simulink model "SWC_FDC_type"  (R2021b)
settings: Solver=FixedStepDiscrete  StartTime=0.0  StopTime=10.0  FixedStep=0.001  RelTol=1e-3
values from neighbouring files (symbols this model uses):
  DID_VCUKey = uint16(0x0202)    [vcu_local_hdr.m]
  DID_XWD = uint16(513)    [vcu_local_hdr.m]
  DIDLen_APSFunConfig = uint16(16)    [vcu_local_hdr.m]
  DIDLen_AutoLock = uint16(1)    [vcu_local_hdr.m]
  DIDLen_DKCKey = uint16(8)    [vcu_local_hdr.m]
  DIDLen_DRLDis = uint16(1)    [vcu_local_hdr.m]
  DIDLen_DynoMode = uint16(1)    [vcu_local_hdr.m]
  DIDLen_FMHTimer = uint16(1)    [vcu_local_hdr.m]
  DIDLen_LFLowPresThre = uint16(1)    [vcu_local_hdr.m]
  DIDLen_LFSensorID = uint16(4)    [vcu_local_hdr.m]
  DIDLen_LRLowPresThre = uint16(1)    [vcu_local_hdr.m]
  DIDLen_LRSensorID = uint16(4)    [vcu_local_hdr.m]
  DIDLen_RFLowPresThre = uint16(1)    [vcu_local_hdr.m]
  DIDLen_RFSensorID = uint16(4)    [vcu_local_hdr.m]
  DIDLen_RRLowPresThre = uint16(1)    [vcu_local_hdr.m]
  DIDLen_RRSensorID = uint16(4)    [vcu_local_hdr.m]
  DIDLen_SensorMode = uint16(1)    [vcu_local_hdr.m]
  DIDLen_TireSize = uint16(16)    [vcu_local_hdr.m]
  DIDLen_TPMSLearnSta = uint16(1)    [vcu_local_hdr.m]
  DIDLen_TurnLampFLThreCurr = uint16(1)    [vcu_local_hdr.m]
  DIDLen_TurnLampFRThreCurr = uint16(1)    [vcu_local_hdr.m]
  DIDLen_TurnLampRLThreCurr = uint16(1)    [vcu_local_hdr.m]
  DIDLen_TurnLampRRThreCurr = uint16(1)    [vcu_local_hdr.m]
  DIDLen_USSConfig = uint16(16)    [vcu_local_hdr.m]
  DIDLen_WhlPres = uint16(4)    [vcu_local_hdr.m]
  DIDLen_WhlSensorBattSta = uint16(1)    [vcu_local_hdr.m]
  DIDLen_WhlTmp = uint16(4)    [vcu_local_hdr.m]
  DIDLen_XWDMode = uint16(1)    [vcu_local_hdr.m]
  DIDNum_APSFunConfig = uint16(0x0903)    [vcu_local_hdr.m]
  DIDNum_AutoLock = uint16(0x0306)    [vcu_local_hdr.m]
  DIDNum_DKCKey = uint16(0x0202)    [vcu_local_hdr.m]
  DIDNum_DRLDis = uint16(0x0307)    [vcu_local_hdr.m]
  DIDNum_DynoMode = uint16(0x0203)    [vcu_local_hdr.m]
  DIDNum_FMHTimer = uint16(0x0305)    [vcu_local_hdr.m]
  DIDNum_LFLowPresThre = uint16(0x0B08)    [vcu_local_hdr.m]
  DIDNum_LFSensorID = uint16(0x0B01)    [vcu_local_hdr.m]
  DIDNum_LRLowPresThre = uint16(0x0B0A)    [vcu_local_hdr.m]
  DIDNum_LRSensorID = uint16(0x0B03)    [vcu_local_hdr.m]
  DIDNum_RFLowPresThre = uint16(0x0B09)    [vcu_local_hdr.m]
  DIDNum_RFSensorID = uint16(0x0B02)    [vcu_local_hdr.m]
  DIDNum_RRLowPresThre = uint16(0x0B0B)    [vcu_local_hdr.m]
  DIDNum_RRSensorID = uint16(0x0B04)    [vcu_local_hdr.m]
  DIDNum_SensorMode = uint16(0x0B0C)    [vcu_local_hdr.m]
  DIDNum_TireSize = uint16(0x0902)    [vcu_local_hdr.m]
  DIDNum_TPMSLearnSta = uint16(0x0B0D)    [vcu_local_hdr.m]
  DIDNum_TurnLampFLThreCurr = uint16(0x0303)    [vcu_local_hdr.m]
  DIDNum_TurnLampFRThreCurr = uint16(0x0301)    [vcu_local_hdr.m]
  DIDNum_TurnLampRLThreCurr = uint16(0x0304)    [vcu_local_hdr.m]
  DIDNum_TurnLampRRThreCurr = uint16(0x0302)    [vcu_local_hdr.m]
  DIDNum_USSConfig = uint16(0x0901)    [vcu_local_hdr.m]
  DIDNum_WhlPres = uint16(0x0B05)    [vcu_local_hdr.m]
  DIDNum_WhlSensorBattSta = uint16(0x0B07)    [vcu_local_hdr.m]
  DIDNum_WhlTmp = uint16(0x0B06)    [vcu_local_hdr.m]
  DIDNum_XWDMode = uint16(0x0201)    [vcu_local_hdr.m]
  DIDVCUKeyLength = uint16(8)    [vcu_local_hdr.m]
  ENUM_DRIVETRAIN_AWD = uint8(  2  )    [vcu_local_hdr.m]
  ENUM_DRIVETRAIN_FWD = uint8(  1  )    [vcu_local_hdr.m]
  ENUM_DRIVETRAIN_RWD = uint8(  0  )    [vcu_local_hdr.m]
  ENUM_TPMSLearnStatus_LEARNED = uint8(  1  )    [vcu_local_hdr.m]
  ENUM_TPMSLearnStatus_LEARNFAIL = uint8(  2  )    [vcu_local_hdr.m]
  ENUM_TPMSLearnStatus_NOTLEARN = uint8(  0  )    [vcu_local_hdr.m]
  ENUM_TPMSSTA_FAT = uint8(  8  )    [vcu_local_hdr.m]
  ENUM_TPMSSTA_LOWBATTERY = uint8(  2  )    [vcu_local_hdr.m]
  FALSE = boolean( 0 )    [vcu_local_hdr.m]
  ONE_INT = uint8(1)    [vcu_local_hdr.m]
  P_boolean = 0.0    [APPTypes.sldd]
  TRUE = boolean( 1 )    [vcu_local_hdr.m]
  ZERO_FLOAT = single(0)    [vcu_local_hdr.m]
  ZERO_INT = uint8(0)    [vcu_local_hdr.m]
undefined symbols (not defined in the file or in its folder): f32_ApsOutVehSpdSig, KHAL_DKCDecryptEnable_flg_ovrdflg, KHAL_DKCDecryptEnable_flg_ovrdval, KHAL_RandomNumberY1_enum, KHAL_RandomNumberY2_enum, KHAL_RandomNumberY_ovrdflg, KHAL_TPMSRESBUTT_flg_ovrdflg, KHAL_TPMSRESBUTT_flg_ovrdval, R_DIDWriteCDD_CSOP_DIDSet_APSFunConfig, R_DIDWriteCDD_CSOP_DIDSet_AutoLock, R_DIDWriteCDD_CSOP_DIDSet_DKCKey, R_DIDWriteCDD_CSOP_DIDSet_DRLDis, R_DIDWriteCDD_CSOP_DIDSet_DynoMode, R_DIDWriteCDD_CSOP_DIDSet_FMHTimer, R_DIDWriteCDD_CSOP_DIDSet_LFLowPresThre, R_DIDWriteCDD_CSOP_DIDSet_LFSensorID, R_DIDWriteCDD_CSOP_DIDSet_LRLowPresThre, R_DIDWriteCDD_CSOP_DIDSet_LRSensorID, R_DIDWriteCDD_CSOP_DIDSet_RFLowPresThre, R_DIDWriteCDD_CSOP_DIDSet_RFSensorID, R_DIDWriteCDD_CSOP_DIDSet_RRLowPresThre, R_DIDWriteCDD_CSOP_DIDSet_RRSensorID, R_DIDWriteCDD_CSOP_DIDSet_SensorMode, R_DIDWriteCDD_CSOP_DIDSet_TireSize, R_DIDWriteCDD_CSOP_DIDSet_TPMSLearnSta, R_DIDWriteCDD_CSOP_DIDSet_TurnLampFLThreCurr, R_DIDWriteCDD_CSOP_DIDSet_TurnLampFRThreCurr, R_DIDWriteCDD_CSOP_DIDSet_TurnLampRLThreCurr, R_DIDWriteCDD_CSOP_DIDSet_TurnLampRRThreCurr, R_DIDWriteCDD_CSOP_DIDSet_USSConfig, R_DIDWriteCDD_CSOP_DIDSet_WhlPres, R_DIDWriteCDD_CSOP_DIDSet_WhlSensorBattSta, R_DIDWriteCDD_CSOP_DIDSet_WhlTmp, R_DIDWriteCDD_CSOP_DIDSet_XWDMode, R_E2E_CAN3_VCU1_CSOP_Write_CAN3_VCU1, R_E2E_CAN3_VCU1_toNIDEC_CSOP_Write_CAN3_VCU1_toNIDEC, R_E2E_CAN4_VCU1_CSOP_Write_CAN4_VCU1, R_FDCCDD_Inner_CSOP_FDC_AppCallSleep, R_HALINCDD_CSOP_PAS_Handler, R_HALINCDD_CSOP_UDS_Main, R_HALOUT_APS_CSOP_ApsOutput, R_HALOUTCDD_CSOP_AppNmStateReq, R_HALOUTCDD_CSOP_SetAcoreRebootCmdACK, R_HALOUTCDD_CSOP_SetSysPwrStat, R_HALOUTCDD_CSOP_SleepRequest, R_IOExpOUT_CDD_CSOP_IOExpSetVal, R_J1939_CAN1_CFGEM1_BAM_CSOP_Write_CAN1_CFGEM1_BAM, R_J1939_CAN1_CFGEM1_DT_CSOP_Write_CAN1_CFGEM1_DT, R_NVMReadCDD_Inner_NVM_ReadOperation, R_NVMWriteCDD_Inner_NVM_WriteOperation, R_UDSCDD_CSOP_DdmRestartOperationCycle, R_WDGCDD_CSOP_Call_Watchdog, R_WDGCDD_CSOP_Call_WDG_AppEnd, R_WDGCDD_CSOP_Call_WDG_AppStart, u16_DIDLen_APSFunConfig, u16_DIDLen_AutoLock, u16_DIDLen_DKCKey, u16_DIDLen_DRLDis, u16_DIDLen_DynoMode, u16_DIDLen_FMHTimer ... (+83)
libraries: simulink x215, FVT_lib x143, hcu_lib x19, hdlsllib x9, app x1, halin x1, halout x1, inp x1, outp x1
(part 2 of 13)

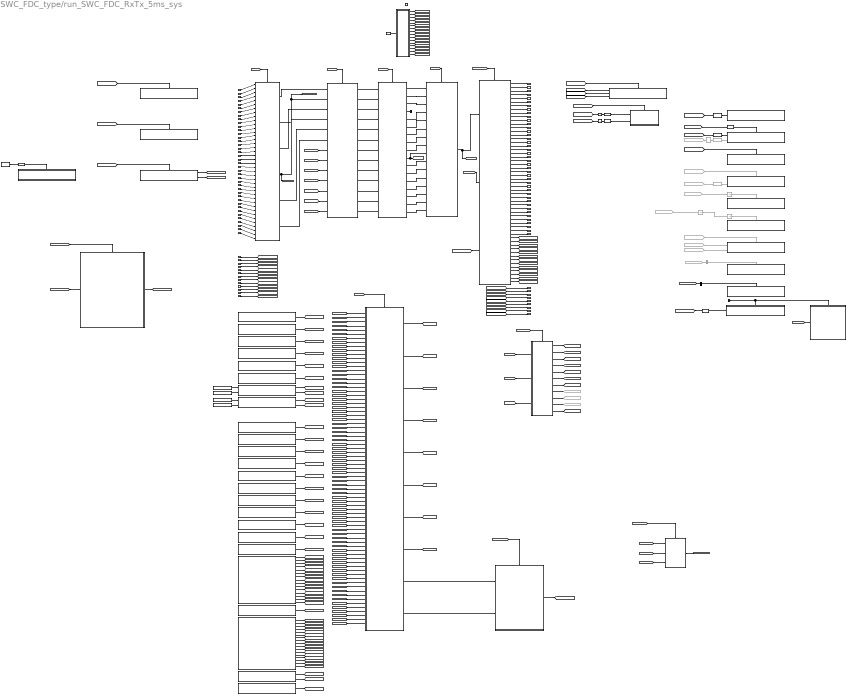
== system SWC_FDC_type/run_SWC_FDC_RxTx_5ms_sys ==
  R_CAN1_DCDC_Status_1_CAN1_SG_DCDC_Status_1_read : Inport
  R_CAN1_DCDC_Status_2_CAN1_SG_DCDC_Status_2_read : Inport  Port=2
  R_CAN1_EAC_Status_1_CAN1_SG_EAC_Status_1_read : Inport  Port=3
  R_CAN1_EBC1_CAN1_SG_EBC1_read : Inport  Port=4
  R_CAN1_EBC2_CAN1_SG_EBC2_read : Inport  Port=5
  R_CAN1_EBC5_CAN1_SG_EBC5_read : Inport  Port=6
  R_CAN1_EHPS_Status_1_CAN1_SG_EHPS_Status_1_read : Inport  Port=7
  R_CAN1_EMC1_EM1_CAN1_SG_EMC1_EM1_read : Inport  Port=8
  R_CAN1_EPB1_CAN1_SG_EPB1_read : Inport  Port=9
  R_CAN1_PDU_Status_1_CAN1_SG_PDU_Status_1_read : Inport  Port=10
  R_CAN2_IVI1_CAN2_SG_IVI1_read : Inport  Port=11
  R_CAN2_IVI2_CAN2_SG_IVI2_read : Inport  Port=12
  R_CAN2_IVI_P20_0_CAN2_SG_IVI_P20_0_read : Inport  Port=13
  R_CAN2_METER1_CAN2_SG_METER1_read : Inport  Port=14
  R_CAN3_BMS1_CAN3_SG_BMS1_read : Inport  Port=15
  R_CAN3_BMS3_CAN3_SG_BMS3_read : Inport  Port=16
  R_CAN3_BMS4_CAN3_SG_BMS4_read : Inport  Port=17
  R_CAN3_BMS5_CAN3_SG_BMS5_read : Inport  Port=18
  R_CAN3_BMS6_CAN3_SG_BMS6_read : Inport  Port=19
  R_CAN3_BMS8_CAN3_SG_BMS8_read : Inport  Port=20
  R_CAN3_CCU1_CAN3_SG_CCU1_read : Inport  Port=21
  R_CAN3_CCU2_CAN3_SG_CCU2_read : Inport  Port=22
  R_CAN3_MCU_B_R1_CAN3_SG_MCU_B_R1_read : Inport  Port=23
  R_CAN3_MCU_B_R2_CAN3_SG_MCU_B_R2_read : Inport  Port=24
  R_CAN3_Shifter1_CAN3_SG_Shifter1_read : Inport  Port=25
  R_CAN4_DKC1_CAN4_SG_DKC1_read : Inport  Port=26
  R_CAN4_DKC2_CAN4_SG_DKC2_read : Inport  Port=27
  R_CAN4_Z24_C1000_0_CAN4_SG_Z24_C1000_0_read : Inport  Port=28
  R_CAN4_Z24_CE100_0_CAN4_SG_Z24_CE100_0_read : Inport  Port=29
  R_CAN4_ZONE_DR1_CAN4_SG_ZONE_DR1_read : Inport  Port=30
  R_CAN4_ZONE_DR_VCU_CAN4_SG_ZONE_DR_VCU_read : Inport  Port=31
  R_CAN4_ZONE_FR1_CAN4_SG_ZONE_FR1_read : Inport  Port=32
  R_CAN4_ZONE_FR_VCU_CAN4_SG_ZONE_FR_VCU_read : Inport  Port=33
  R_CAN4_zGW_APTC1_CAN4_SG_zGW_APTC1_read : Inport  Port=34
  R_CAN4_zGW_CANFr1_CAN4_SG_zGW_CANFr1_read : Inport  Port=35
  R_CAN4_zGW_LINDr1_CAN4_SG_zGW_LINDr1_read : Inport  Port=36
  R_CAN5_TBOX1_CAN5_SG_TBOX1_read : Inport  Port=37
  R_CAN5_TBOX2_CAN5_SG_TBOX2_read : Inport  Port=38
  R_CAN5_TBOX3_CAN5_SG_TBOX3_read : Inport  Port=39
  R_CAN7_Door_Fr1_CAN7_SG_Door_Fr1_read : Inport  Port=40
  IRV_u16Array4_ApsInDist_read : Inport  Port=41
  IRV_u8Array12_ApsInUssSta_read : Inport  Port=42
  IRV_u8Array256_NvmReadArray_read : Inport  Port=43
  IRV_u8Array8_ApsInLevel_read : Inport  Port=44
  IRV_u8Array8_PasInDist_read : Inport  Port=45
  IRV_u8Array9_TPMSData_read : Inport  Port=46
  IRV_u8_ApsInPASChime_read : Inport  Port=47
  IRV_u8_ApsInSensorLayout_read : Inport  Port=48
  IRV_u8_ApsInSysFailSta_read : Inport  Port=49
  IRV_u8_ApsInSysMode_read : Inport  Port=50
  IRV_u8_CTDSW_read : Inport  Port=51
  IRV_u8_TPMSDataInSta_read : Inport  Port=52
  IRV_u8_TrunkHanSW_read : Inport  Port=53
  function : TriggerPort  TriggerType=function-call  VariantControl=(inherit)  SampleTimeType=periodic  SampleTime=-1
  APP : app/APP  SystemSampleTime=-1  VariantActivationTime=update diagram  Latency=0  AutoFrameSizeCalculation=off
  Bus Selector : BusSelector  Commented=on  OutputSignals=VOUTP_EnterNewOperCyc_flg
  Bus Selector1 : BusSelector  OutputSignals=VOUTP_AcoreRebootCmdACK_flg
  Cast To Boolean : DataTypeConversion  OutDataTypeStr=boolean
  Cast To Boolean1 : DataTypeConversion  OutDataTypeStr=boolean
  Constant : Constant  Value=DIDVCUKeyLength
  Constant1 : Constant  Value=DID_VCUKey
  Constant2 : Constant  Value=uint16(ONE_INT)
  Constant3 : Constant  Value=DID_XWD
  Constant4 : Constant  Value=TRUE
  Constant5 : Constant  Value=FALSE
  Constant6 : Constant  Value=ONE_INT
  Data Type Conversion : DataTypeConversion  OutDataTypeStr=uint8
  Data Type Conversion1 : DataTypeConversion  OutDataTypeStr=uint8
  Data Type Conversion2 : DataTypeConversion  Commented=on  OutDataTypeStr=uint8
  Data Type Conversion3 : DataTypeConversion  Commented=on  OutDataTypeStr=uint32
  Data Type Conversion5 : DataTypeConversion  OutDataTypeStr=uint8
  From11 : From  Commented=on  GotoTag=VOUTP_NetworkReq_flg
  From129 : From  Commented=on  GotoTag=BOUTP_outputs
  From14 : From  Commented=on  GotoTag=VOUTP_FdcSlpTime_sec
  From15 : From  Commented=on  GotoTag=VOUTP_FdcSlpReqRisingEdge_flg
  From16 : From  Commented=on  GotoTag=VOUTP_FdcSlpReqRisingEdge_flg
  From17 : From  Commented=on  GotoTag=VOUTP_FdcSlpReqRisingEdge_flg
  From18 : From  Commented=on  GotoTag=Header_Array
  From19 : From  Commented=on  GotoTag=DTC_Array
  From20 : From  Commented=on  GotoTag=DTC_Trigger
  Goto103 : Goto  Commented=on  GotoTag=Header_Array
  Goto108 : Goto  Commented=on  GotoTag=DTC_Array
  Goto116 : Goto  Commented=on  GotoTag=DTC_Trigger
  Ground10 : Ground
  HALOUT_AFTER : Subsystem
  HAL_IN : halin/HAL_IN  SystemSampleTime=-1  VariantActivationTime=update diagram  Latency=0  AutoFrameSizeCalculation=off
  HAL_OUT : halout/HAL_OUT  SystemSampleTime=-1  VariantActivationTime=update diagram  Latency=0  AutoFrameSizeCalculation=off
  Halin_CDD : Subsystem
      settings: RTWSystemCode=Nonreusable function  RTWFcnNameOpts=Use subsystem name  RTWFileNameOpts=Use subsystem name
  INP : inp/INP  SystemSampleTime=-1  VariantActivationTime=update diagram  Latency=0  AutoFrameSizeCalculation=off
  NOT : Logic  Commented=on  Operator=NOT  Inputs=1  AllPortsSameDT=off  OutDataTypeStr=boolean
  OUTP : outp/OUTP  SystemSampleTime=-1  VariantActivationTime=update diagram  Latency=0  AutoFrameSizeCalculation=off
  OUTP_AFTER : Subsystem
      settings: RTWSystemCode=Nonreusable function  RTWFcnNameOpts=Use subsystem name  RTWFileNameOpts=Use subsystem name
  R_FDCCDD_Inner_CSOP_FDC_AppCallSleep : Subsystem
  R_HALINCDD_CSOP_AnyNmID : FunctionCaller  FunctionPrototype=u8_AnyNMID = R_HALINCDD_CSOP_AnyNmID()  OutputArgumentSpecifications=uint8(1)
  R_HALINCDD_CSOP_CAN1BusOff : FunctionCaller  FunctionPrototype=u8_CAN1BusOff = R_HALINCDD_CSOP_CAN1BusOff()  OutputArgumentSpecifications=uint8(1)
  R_HALINCDD_CSOP_CAN2BusOff : FunctionCaller  FunctionPrototype=u8_CAN2BusOff = R_HALINCDD_CSOP_CAN2BusOff()  OutputArgumentSpecifications=uint8(1)
  R_HALINCDD_CSOP_CAN3BusOff : FunctionCaller  FunctionPrototype=u8_CAN3BusOff = R_HALINCDD_CSOP_CAN3BusOff()  OutputArgumentSpecifications=uint8(1)
  R_HALINCDD_CSOP_CAN4BusOff : FunctionCaller  FunctionPrototype=u8_CAN4BusOff = R_HALINCDD_CSOP_CAN4BusOff()  OutputArgumentSpecifications=uint8(1)
  R_HALINCDD_CSOP_CAN5BusOff : FunctionCaller  FunctionPrototype=u8_CAN5BusOff = R_HALINCDD_CSOP_CAN5BusOff()  OutputArgumentSpecifications=uint8(1)
  R_HALINCDD_CSOP_DIDgetDKCdata : FunctionCaller  FunctionPrototype=[u8_DidStaDKC,u8Array8_DidDataDKC] = R_HALINCDD_CSOP_DIDgetDKCdata(u16_lengthDIDDKC,u16_DIDDKC)  InputArgumentSpecifications=uint16(1), uint16(1)  OutputArgumentSpecifications=uint8(1), uint8([1;1;1;1;1;1;1;1])
  R_HALINCDD_CSOP_DIDgetXWDdata : FunctionCaller  FunctionPrototype=[u8_DidStaXWD,u8_DidDataXWD] = R_HALINCDD_CSOP_DIDgetXWDdata(u16_lengthDIDXWD,u16_DIDXWD)  InputArgumentSpecifications=uint16(1), uint16(1)  OutputArgumentSpecifications=uint8(1), uint8(1)
  R_HALINCDD_CSOP_GetAcoreReadyToSleep : FunctionCaller  FunctionPrototype=s8_AcoreReadyToSleep = R_HALINCDD_CSOP_GetAcoreReadyToSleep()  OutputArgumentSpecifications=int8(1)
  R_HALINCDD_CSOP_GetAcoreRebootCmd : FunctionCaller  FunctionPrototype=u8_AcoreRebootCmd = R_HALINCDD_CSOP_GetAcoreRebootCmd()  OutputArgumentSpecifications=uint8(1)
  R_HALINCDD_CSOP_GetAuxBattVoltage : FunctionCaller  FunctionPrototype=u16_AuxBattVol100mV = R_HALINCDD_CSOP_GetAuxBattVoltage()  OutputArgumentSpecifications=uint16(1)
  R_HALINCDD_CSOP_GetBootReason : FunctionCaller  FunctionPrototype=u8_BootReason = R_HALINCDD_CSOP_GetBootReason()  OutputArgumentSpecifications=uint8(1)
  R_HALINCDD_CSOP_GetEvccAplusPwrUpReq : FunctionCaller  FunctionPrototype=u8_EvccAplusPwrUpReq = R_HALINCDD_CSOP_GetEvccAplusPwrUpReq()  OutputArgumentSpecifications=uint8(1)
  R_HALINCDD_CSOP_GetNmState : FunctionCaller  FunctionPrototype=u8_CurrentNMState = R_HALINCDD_CSOP_GetNmState()  OutputArgumentSpecifications=uint8(1)
  R_HALINCDD_CSOP_GetNvmProtectState : FunctionCaller  FunctionPrototype=u8_NvmProtectSta = R_HALINCDD_CSOP_GetNvmProtectState()  OutputArgumentSpecifications=uint8(1)
  R_HALINCDD_CSOP_GetSWID : FunctionCaller  FunctionPrototype=u8Array30_SWID = R_HALINCDD_CSOP_GetSWID()  OutputArgumentSpecifications=uint8([1;1;1;1;1;1;1;1;1;1;1;1;1;1;1;1;1;1;1;1;1;1;1;1;1;1;1;1;1;1])
  R_HALINCDD_CSOP_GetVinpAllowMoveThdOta : FunctionCaller  FunctionPrototype=u8_AllowMovThdOTA = R_HALINCDD_CSOP_GetVinpAllowMoveThdOta()  OutputArgumentSpecifications=uint8(1)
  R_HALINCDD_CSOP_GetVinpPwrReqOta : FunctionCaller  FunctionPrototype=u8_PwrReqOTA = R_HALINCDD_CSOP_GetVinpPwrReqOta()  OutputArgumentSpecifications=uint8(1)
  R_HALINCDD_CSOP_GetWISR : FunctionCaller  FunctionPrototype=u32_WISR = R_HALINCDD_CSOP_GetWISR()  OutputArgumentSpecifications=uint32(1)
  R_HALINCDD_CSOP_HALINCDD_DIRECT : FunctionCaller  FunctionPrototype=[u8_BrakeSW,u8_BrakeLamp,u16_Pedal1Vol,u16_Pedal2Vol,u16_Pedal1Ref5V,u16_Pedal2Ref5V,u8_DrDoorSW,u8_PsDoorSW,u8_RRDoorSW,u8_RLDoorSW,u8_HoodSW,u8_TailgateSW,u8_HazardSW,u8_SeatSW,u8_CrashSignal] = R_HALINCDD_CSOP_HALINCDD_DIRECT()  OutputArgumentSpecifications=uint8(1), uint8(1), uint16(1), uint16(1), uint16(1), uint16(1), uint8(1), uint8(1), uint8(1), uint8(1), uint8(1), uint8(1), uint8(1), uint8(1), uint8(1)
  R_HALINCDD_u8Array4_HWID : FunctionCaller  FunctionPrototype=u8Array4_HWID = R_HALINCDD_u8Array4_HWID()  OutputArgumentSpecifications=uint8([1;1;1;1])
  R_HALIN_APS_CSOP_ApsGetData : FunctionCaller  FunctionPrototype=[u8_GetAPS_Progress_PCT,u8_GetAPS_RQ_Display,u8_GetAPS_SW_Ver,u8_GetAPS_HW_Ver,u8_GetAPS_ExitCondition,f32_GetAPS_Angle_Target,u8_GetAPS_Sta_System,u8_GetAPS_V_Rq_EPAS_Ctrl,u8_GetAPS_Rq_EPAS_Ctrl,u8_GetAPS_Req,f32_GetAPS_DecReq,u8_GetAPS_DecReq_A,f32_GetAPS_SpeedCmd,u8_GetAPS_ShftPosnReq,u8_GetAPS_VMC_Req_A,u8_GetCAAS_Sta,u8_GetCAAS_VMC_Req_A] = R_HALIN_APS_CSOP_ApsGetData()  OutputArgumentSpecifications=uint8(1), uint8(1), uint8(1), uint8(1), uint8(1), single(1), uint8(1), uint8(1), uint8(1), uint8(1), single(1), uint8(1), single(1), uint8(1), uint8(1), uint8(1), uint8(1)
  R_HALIN_IMU_CSOP_IMUGetOffsetVal : Subsystem
  R_HALIN_IMU_CSOP_IMUGetSixAxisVal : FunctionCaller  FunctionPrototype=[s16_IMUSixAxisVal,u8_IMUSixAxisValSta] = R_HALIN_IMU_CSOP_IMUGetSixAxisVal()  OutputArgumentSpecifications=int16([1;1;1;1;1;1]), uint8(1)
  R_HALOUTCDD_CSOP_AppNmStateReq : Subsystem
  R_HALOUTCDD_CSOP_SetAcoreRebootCmdACK : Subsystem
  R_HALOUTCDD_CSOP_SetSysPwrStat : FunctionCaller  FunctionPrototype=R_HALOUTCDD_CSOP_SetSysPwrStat(u8_SysPwrStat)  InputArgumentSpecifications=uint8(1)
  R_HALOUTCDD_CSOP_SleepRequest : Subsystem
  R_NVMReadCDD_Inner_NVM_ReadOperation : Subsystem
  R_NVMWriteCDD_Inner_NVM_WriteOperation : Subsystem
  R_UDSCDD_CSOP_DdmClearDTCNotification : FunctionCaller  FunctionPrototype=u8_ClearDTCcmd = R_UDSCDD_CSOP_DdmClearDTCNotification()  OutputArgumentSpecifications=uint8(1)
  R_UDSCDD_CSOP_DdmRestartOperationCycle : Subsystem
  R_UDSCDD_CSOP_SetDTCStatus : Subsystem
  R_WDGCDD_CSOP_Call_WDG_AppEnd : Subsystem
  R_WDGCDD_CSOP_Call_WDG_AppStart : Subsystem
  R_WDGCDD_CSOP_Call_Watchdog : Subsystem
  Subsystem : Subsystem
  Subsystem1 : Subsystem
  Subsystem2 : Subsystem
  Subsystem3 : Subsystem
  Subsystem4 : Subsystem
  Subsystem5 : Subsystem
  Terminator : Terminator
  Unit Delay : UnitDelay  Commented=on  SampleTime=-1  HasFrameUpgradeWarning=on
  Unit Delay1 : UnitDelay  Commented=on  SampleTime=-1  HasFrameUpgradeWarning=on
  Unit Delay2 : UnitDelay  Commented=on  SampleTime=-1  HasFrameUpgradeWarning=on
  Unit Delay4 : UnitDelay  SampleTime=-1  HasFrameUpgradeWarning=on
  Unit Delay5 : UnitDelay  SampleTime=-1  HasFrameUpgradeWarning=on
  detect_Increase : simulink/Logic and Bit Operations/Detect Increase  vinit=0.0  OutDataTypeStr=boolean
  detect_change : simulink/Logic and Bit Operations/Detect Change  vinit=0  OutDataTypeStr=boolean
  hcu_main_sched : Stateflow chart  TreatAsAtomicUnit=on
  P_CAN1_GW1_C1000_1_CAN1_SG_GW1_C1000_1_write : Outport
  P_CAN2_FD2_CE100_0_CAN2_SG_FD2_CE100_0_write : Outport  Port=2
  P_CAN2_FD2_CE100_1_CAN2_SG_FD2_CE100_1_write : Outport  Port=3
  P_CAN2_FD2_CE200_1_CAN2_SG_FD2_CE200_1_write : Outport  Port=4
  P_CAN3_FD3_BCM1_CAN3_SG_FD3_BCM1_write : Outport  Port=5
  P_CAN3_FD3_THCM2_CAN3_SG_FD3_THCM2_write : Outport  Port=6
  P_CAN3_FD3_V2L1_CAN3_SG_FD3_V2L1_write : Outport  Port=7
  P_CAN3_GW3_CE100_0_CAN3_SG_GW3_CE100_0_write : Outport  Port=8
  P_CAN4_FD4_CE100_1_CAN4_SG_FD4_CE100_1_write : Outport  Port=9
  P_CAN4_FD4_CE100_3_CAN4_SG_FD4_CE100_3_write : Outport  Port=10
  P_CAN4_FD4_CE200_0_CAN4_SG_FD4_CE200_0_write : Outport  Port=11
  P_CAN4_GW4_CE100_0_CAN4_SG_GW4_CE100_0_write : Outport  Port=12
  P_CAN5_FD5_CE100_0_CAN5_SG_FD5_CE100_0_write : Outport  Port=13
  P_CAN5_FD5_Debug1_CAN5_SG_FD5_Debug1_write : Outport  Port=14
  P_CAN5_GW5_CE100_0_CAN5_SG_GW5_CE100_0_write : Outport  Port=15
  P_CAN7_FD7_CE100_0_CAN7_SG_FD7_CE100_0_write : Outport  Port=16
  P_CAN7_FD7_CE100_1_CAN7_SG_FD7_CE100_1_write : Outport  Port=17
  IRV_ms10_CAN1_SG_EMRC1_write : Outport  Port=18  OutDataTypeStr=Bus: DT_CAN1_SG_EMRC1  PortDimensions=1  BusOutputAsStruct=on
  IRV_ms10_CAN1_SG_VCU_PDU_Demand_1_write : Outport  Port=19  OutDataTypeStr=Bus: DT_CAN1_SG_VCU_PDU_Demand_1  PortDimensions=1  BusOutputAsStruct=on
  IRV_ms10_CAN2_SG_GW2_C10_0_write : Outport  Port=20  OutDataTypeStr=Bus: DT_CAN2_SG_GW2_C10_0  PortDimensions=1  BusOutputAsStruct=on
  IRV_ms10_CAN3_SG_FD3_VCU0_write : Outport  Port=21  OutDataTypeStr=Bus: DT_CAN3_SG_FD3_VCU0  PortDimensions=1  BusOutputAsStruct=on
  IRV_ms10_CAN3_SG_FD3_VCU2_write : Outport  Port=22  OutDataTypeStr=Bus: DT_CAN3_SG_FD3_VCU2  PortDimensions=1  BusOutputAsStruct=on
  IRV_ms10_CAN3_SG_FD3_VCU2_toNIDEC_write : Outport  Port=23  OutDataTypeStr=Bus: DT_CAN3_SG_FD3_VCU2_toNIDEC  PortDimensions=1  BusOutputAsStruct=on
  IRV_ms10_CAN3_SG_FD3_VCU5_write : Outport  Port=24  OutDataTypeStr=Bus: DT_CAN3_SG_FD3_VCU5  PortDimensions=1  BusOutputAsStruct=on
  IRV_ms100_CAN1_SG_CCVS_write : Outport  Port=25  OutDataTypeStr=Bus: DT_CAN1_SG_CCVS  PortDimensions=1  BusOutputAsStruct=on
  IRV_ms100_CAN1_SG_FD1_C100_1_write : Outport  Port=26  OutDataTypeStr=Bus: DT_CAN1_SG_FD1_C100_1  PortDimensions=1  BusOutputAsStruct=on
  IRV_ms100_CAN1_SG_FD1_C100_2_write : Outport  Port=27  OutDataTypeStr=Bus: DT_CAN1_SG_FD1_C100_2  PortDimensions=1  BusOutputAsStruct=on
  IRV_ms100_CAN1_SG_FD1_C100_3_write : Outport  Port=28  OutDataTypeStr=Bus: DT_CAN1_SG_FD1_C100_3  PortDimensions=1  BusOutputAsStruct=on
  IRV_ms100_CAN1_SG_FD1_CE100_1_write : Outport  Port=29  OutDataTypeStr=Bus: DT_CAN1_SG_FD1_CE100_1  PortDimensions=1  BusOutputAsStruct=on
  IRV_ms100_CAN1_SG_GW1_C100_4_write : Outport  Port=30  OutDataTypeStr=Bus: DT_CAN1_SG_GW1_C100_4  PortDimensions=1  BusOutputAsStruct=on
  IRV_ms100_CAN2_SG_FD2_C200_1_write : Outport  Port=31  OutDataTypeStr=Bus: DT_CAN2_SG_FD2_C200_1  PortDimensions=1  BusOutputAsStruct=on
  IRV_ms100_CAN3_SG_FD3_THCM1_write : Outport  Port=32  OutDataTypeStr=Bus: DT_CAN3_SG_FD3_THCM1  PortDimensions=1  BusOutputAsStruct=on
  IRV_ms100_CAN4_SG_FD4_C100_0_write : Outport  Port=33  OutDataTypeStr=Bus: DT_CAN4_SG_FD4_C100_0  PortDimensions=1  BusOutputAsStruct=on
  IRV_ms20_CAN2_SG_FD2_C20_0_write : Outport  Port=34  OutDataTypeStr=Bus: DT_CAN2_SG_FD2_C20_0  PortDimensions=1  BusOutputAsStruct=on
  IRV_ms250_CAN1_SG_EEC3_write : Outport  Port=35  OutDataTypeStr=Bus: DT_CAN1_SG_EEC3  PortDimensions=1  BusOutputAsStruct=on
  IRV_ms50_CAN1_SG_EEC2_write : Outport  Port=36  OutDataTypeStr=Bus: DT_CAN1_SG_EEC2  PortDimensions=1  BusOutputAsStruct=on
  IRV_ms50_CAN1_SG_ETC2_write : Outport  Port=37  OutDataTypeStr=Bus: DT_CAN1_SG_ETC2  PortDimensions=1  BusOutputAsStruct=on
  IRV_ms5000_CAN2_SG_FD2_Version_write : Outport  Port=38  OutDataTypeStr=Bus: DT_CAN2_SG_FD2_Version  PortDimensions=1  BusOutputAsStruct=on
  IRV_ms80_CAN1_SG_ETC1_write : Outport  Port=39  OutDataTypeStr=Bus: DT_CAN1_SG_ETC1  PortDimensions=1  BusOutputAsStruct=on
  IRV_E2E_CAN3_SG_FD3_VCU1_write : Outport  Port=40  OutDataTypeStr=Bus: DT_CAN3_SG_FD3_VCU1  PortDimensions=1  BusOutputAsStruct=on
  IRV_E2E_CAN3_SG_FD3_VCU1_toNIDEC_write : Outport  Port=41  OutDataTypeStr=Bus: DT_CAN3_SG_FD3_VCU1_toNIDEC  PortDimensions=1  BusOutputAsStruct=on
  IRV_E2E_CAN4_SG_FD4_CE100_0_write : Outport  Port=42  OutDataTypeStr=Bus: DT_CAN4_SG_FD4_CE100_0  PortDimensions=1  BusOutputAsStruct=on
  IRV_J1939_CAN1_SG_CFGEM1_BAM_write : Outport  Port=43  OutDataTypeStr=Bus: DT_CAN1_SG_CFGEM1_BAM  PortDimensions=1  BusOutputAsStruct=on
  IRV_J1939_CAN1_SG_CFGEM1_DT_write : Outport  Port=44  OutDataTypeStr=Bus: DT_CAN1_SG_CFGEM1_DT  PortDimensions=1  BusOutputAsStruct=on
  IRV_f32_ApsOutVehSpdSig_write : Outport  Port=45  OutDataTypeStr=single  PortDimensions=1
  IRV_u8Array256_NvmWriteArray_write : Outport  Port=46  OutDataTypeStr=uint8  PortDimensions=256
  IRV_u8_ApsOutGearPosnSig_write : Outport  Port=47  OutDataTypeStr=uint8  PortDimensions=1
  IRV_u8_ApsOutSendChrgPlugSta_write : Outport  Port=48  OutDataTypeStr=uint8  PortDimensions=1
  IRV_u8_ApsOutSetFrSensorOnCmd_write : Outport  Port=49  OutDataTypeStr=uint8  PortDimensions=1
  IRV_u8_ApsOutSetFrSensorSwTOCmd_write : Outport  Port=50  OutDataTypeStr=uint8  PortDimensions=1
  IRV_u8_ApsOutSetVehSpdTOCmd_write : Outport  Port=51  OutDataTypeStr=uint8  PortDimensions=1
  wires:
  IRV_u16Array4_ApsInDist_read/1 -> [u16Array4_ApsInDist]
  IRV_u8Array12_ApsInUssSta_read/1 -> [u8Array12_ApsInUssSta]
  IRV_u8Array256_NvmReadArray_read/1 -> [u8Array256_NvmReadArray]
  IRV_u8Array8_ApsInLevel_read/1 -> [u8Array8_ApsInLevel]
  IRV_u8Array8_PasInDist_read/1 -> [u8Array8_PasInDist]
  IRV_u8Array9_TPMSData_read/1 -> [u8Array9_TPMSData]
  IRV_u8_ApsInPASChime_read/1 -> [u8_ApsInPASChime]
  IRV_u8_ApsInSensorLayout_read/1 -> [u8_ApsInSensorLayout]
  IRV_u8_ApsInSysFailSta_read/1 -> [u8_ApsInSysFailSta]
  IRV_u8_ApsInSysMode_read/1 -> [u8_ApsInSysMode]
  IRV_u8_CTDSW_read/1 -> [u8_CTDSW]
  IRV_u8_TPMSDataInSta_read/1 -> [u8_TPMSDataInSta]
  IRV_u8_TrunkHanSW_read/1 -> [u8_TrunkHanSW]
  [J1939_CAN1_SG_CFGEM1_BAM] -> IRV_J1939_CAN1_SG_CFGEM1_BAM_write/1
  [J1939_CAN1_SG_CFGEM1_DT] -> IRV_J1939_CAN1_SG_CFGEM1_DT_write/1
  [f32_ApsOutVehSpdSig] -> IRV_f32_ApsOutVehSpdSig_write/1
  [u8Array256_NvmWriteArray] -> IRV_u8Array256_NvmWriteArray_write/1
  [u8_ApsOutGearPosnSig] -> IRV_u8_ApsOutGearPosnSig_write/1
  [u8_ApsOutSendChrgPlugSta] -> IRV_u8_ApsOutSendChrgPlugSta_write/1
  [u8_ApsOutSetFrSensorOnCmd] -> IRV_u8_ApsOutSetFrSensorOnCmd_write/1
  [u8_ApsOutSetFrSensorSwTOCmd] -> IRV_u8_ApsOutSetFrSensorSwTOCmd_write/1
  [u8_ApsOutSetVehSpdTOCmd] -> IRV_u8_ApsOutSetVehSpdTOCmd_write/1
  R_HALINCDD_CSOP_AnyNmID/1 -> [u8_AnyNMID]
  R_HALINCDD_CSOP_CAN1BusOff/1 -> [u8_CAN1BusOff]
  R_HALINCDD_CSOP_CAN2BusOff/1 -> [u8_CAN2BusOff]
  R_HALINCDD_CSOP_CAN3BusOff/1 -> [u8_CAN3BusOff]
  R_HALINCDD_CSOP_CAN4BusOff/1 -> [u8_CAN4BusOff]
  R_HALINCDD_CSOP_CAN5BusOff/1 -> [u8_CAN5BusOff]
  Constant/1 -> R_HALINCDD_CSOP_DIDgetDKCdata/1
  Constant1/1 -> R_HALINCDD_CSOP_DIDgetDKCdata/2
  R_HALINCDD_CSOP_DIDgetDKCdata/1 -> [u8_DidStaDKC]
  R_HALINCDD_CSOP_DIDgetDKCdata/2 -> [u8Array8_DidDataDKC]
  Constant2/1 -> R_HALINCDD_CSOP_DIDgetXWDdata/1
  Constant3/1 -> R_HALINCDD_CSOP_DIDgetXWDdata/2
  R_HALINCDD_CSOP_DIDgetXWDdata/1 -> [u8_DidStaXWD]
  R_HALINCDD_CSOP_DIDgetXWDdata/2 -> [u8_DidDataXWD]
  R_HALINCDD_CSOP_GetAcoreReadyToSleep/1 -> [s8_AcoreReadyToSleep]
  R_HALINCDD_CSOP_GetAcoreRebootCmd/1 -> [u8_AcoreRebootCmd]
  R_HALINCDD_CSOP_GetAuxBattVoltage/1 -> [u16_AuxBattVol100mV]
  R_HALINCDD_CSOP_GetBootReason/1 -> [u8_BootReason]
  R_HALINCDD_CSOP_GetEvccAplusPwrUpReq/1 -> [u8_EvccAplusPwrUpReq]
  R_HALINCDD_CSOP_GetNmState/1 -> [u8_CurrentNMState]
  R_HALINCDD_CSOP_GetNvmProtectState/1 -> [u8_NvmProtectSta]
  R_HALINCDD_CSOP_GetSWID/1 -> [u8Array30_SWID]
  R_HALINCDD_CSOP_GetVinpAllowMoveThdOta/1 -> [u8_AllowMovThdOTA]
  R_HALINCDD_CSOP_GetVinpPwrReqOta/1 -> [u8_PwrReqOTA]
  R_HALINCDD_CSOP_GetWISR/1 -> [u32_WISR]
  R_HALINCDD_CSOP_HALINCDD_DIRECT/1 -> [u8_BrakeSW]
  R_HALINCDD_CSOP_HALINCDD_DIRECT/2 -> [u8_BrakeLamp]
  R_HALINCDD_CSOP_HALINCDD_DIRECT/3 -> [u16_Pedal1Vol]
  R_HALINCDD_CSOP_HALINCDD_DIRECT/4 -> [u16_Pedal2Vol]
  R_HALINCDD_CSOP_HALINCDD_DIRECT/5 -> [u16_Pedal1Ref5V]
  R_HALINCDD_CSOP_HALINCDD_DIRECT/6 -> [u16_Pedal2Ref5V]
  R_HALINCDD_CSOP_HALINCDD_DIRECT/7 -> [u8_DrDoorSW]
  R_HALINCDD_CSOP_HALINCDD_DIRECT/8 -> [u8_PsDoorSW]
  R_HALINCDD_CSOP_HALINCDD_DIRECT/9 -> [u8_RRDoorSW]
  R_HALINCDD_CSOP_HALINCDD_DIRECT/10 -> [u8_RLDoorSW]
  R_HALINCDD_CSOP_HALINCDD_DIRECT/11 -> [u8_HoodSW]
  R_HALINCDD_CSOP_HALINCDD_DIRECT/12 -> [u8_TailgateSW]
  R_HALINCDD_CSOP_HALINCDD_DIRECT/13 -> [u8_HazardSW]
  R_HALINCDD_CSOP_HALINCDD_DIRECT/14 -> [u8_SeatSW]
  R_HALINCDD_CSOP_HALINCDD_DIRECT/15 -> [u8_CrashSignal]
  R_HALINCDD_u8Array4_HWID/1 -> [u8Array4_HWID]
  R_HALIN_APS_CSOP_ApsGetData/1 -> [u8_GetAPS_Progress_PCT]
  R_HALIN_APS_CSOP_ApsGetData/2 -> [u8_GetAPS_RQ_Display]
  R_HALIN_APS_CSOP_ApsGetData/3 -> [u8_GetAPS_SW_Ver]
  R_HALIN_APS_CSOP_ApsGetData/4 -> [u8_GetAPS_HW_Ver]
  R_HALIN_APS_CSOP_ApsGetData/5 -> [u8_GetAPS_ExitCondition]
  R_HALIN_APS_CSOP_ApsGetData/6 -> [f32_GetAPS_Angle_Target]
  R_HALIN_APS_CSOP_ApsGetData/7 -> [u8_GetAPS_Sta_System]
  R_HALIN_APS_CSOP_ApsGetData/8 -> [u8_GetAPS_V_Rq_EPAS_Ctrl]
  R_HALIN_APS_CSOP_ApsGetData/9 -> [u8_GetAPS_Rq_EPAS_Ctrl]
  R_HALIN_APS_CSOP_ApsGetData/10 -> [u8_GetAPS_Req]
  R_HALIN_APS_CSOP_ApsGetData/11 -> [f32_GetAPS_DecReq]
  R_HALIN_APS_CSOP_ApsGetData/12 -> [u8_GetAPS_DecReq_A]
  R_HALIN_APS_CSOP_ApsGetData/13 -> [f32_GetAPS_SpeedCmd]
  R_HALIN_APS_CSOP_ApsGetData/14 -> [u8_GetAPS_ShftPosnReq]
  R_HALIN_APS_CSOP_ApsGetData/15 -> [u8_GetAPS_VMC_Req_A]
  R_HALIN_APS_CSOP_ApsGetData/16 -> [u8_GetCAAS_Sta]
  R_HALIN_APS_CSOP_ApsGetData/17 -> [u8_GetCAAS_VMC_Req_A]
  R_HALIN_IMU_CSOP_IMUGetSixAxisVal/1 -> [s16_IMUSixAxisVal]
  R_HALIN_IMU_CSOP_IMUGetSixAxisVal/2 -> [u8_IMUSixAxisValSta]
  R_UDSCDD_CSOP_DdmClearDTCNotification/1 -> [u8_ClearDTCcmd]
  Data Type Conversion/1 -> R_HALOUTCDD_CSOP_SetSysPwrStat/1
  [VOUTP_SysPowerMode_enum] -> Data Type Conversion/1
  Data Type Conversion1/1 -> R_HALOUTCDD_CSOP_AppNmStateReq/1(WakeReq)
  [VOUTP_NetworkReq_flg] -> Data Type Conversion1/1
  Data Type Conversion2/1 -> R_HALOUTCDD_CSOP_AppNmStateReq/2(SleepReq)
  NOT/1 -> Data Type Conversion2/1
  From11/1 -> NOT/1
  detect_change/1 -> R_HALOUTCDD_CSOP_AppNmStateReq/Enable
  [VOUTP_NetworkReq_flg] -> detect_change/1
  [VOUTP_NvWriteReqRisingEdge_flg] -> R_NVMWriteCDD_Inner_NVM_WriteOperation/Enable
  Data Type Conversion3/1 -> R_HALOUTCDD_CSOP_SleepRequest/2(WakeUpTime)
  From14/1 -> Data Type Conversion3/1
  From15/1 -> R_HALOUTCDD_CSOP_SleepRequest/Enable
  Unit Delay/1 -> R_WDGCDD_CSOP_Call_WDG_AppEnd/Enable
  From16/1 -> Unit Delay/1
  Unit Delay1/1 -> R_FDCCDD_Inner_CSOP_FDC_AppCallSleep/Enable
  Unit Delay2/1 -> Unit Delay1/1
  From17/1 -> Unit Delay2/1
  From18/1 -> R_UDSCDD_CSOP_SetDTCStatus/1(Header_Array)
  From19/1 -> R_UDSCDD_CSOP_SetDTCStatus/2(DTC_Array)
  From20/1 -> R_UDSCDD_CSOP_SetDTCStatus/Enable
  [trig_Read_NVM_00] -> R_NVMReadCDD_Inner_NVM_ReadOperation/Trigger
  [trig_WDG] -> R_WDGCDD_CSOP_Call_Watchdog/Trigger
  detect_Increase/1 -> R_WDGCDD_CSOP_Call_WDG_AppStart/Enable
  Constant4/1 -> detect_Increase/1
  [trig_ReadIMUOffset_00] -> R_HALIN_IMU_CSOP_IMUGetOffsetVal/Trigger
  R_HALIN_IMU_CSOP_IMUGetOffsetVal/1(Out1) -> [s16_IMUOffsetVal]
  R_HALIN_IMU_CSOP_IMUGetOffsetVal/2(Out2) -> [u8_IMUOffsetValSta]
  [E2E_CAN3_VCU1_Trigger] -> HALOUT_AFTER/1(E2E_CAN3_VCU1_Trigger)
  [E2E_CAN3_VCU1_toNIDEC_Trigger] -> HALOUT_AFTER/2(E2E_CAN3_VCU1_Trigger_toNIDEC)
  [E2E_CAN4_VCU1_Trigger] -> HALOUT_AFTER/3(E2E_CAN4_VCU1_Trigger)
  [trig_HAL_OUTAFTER_50_1] -> HALOUT_AFTER/Trigger
  INP/5 -> APP/5
  INP/1 -> APP/1
  hcu_main_sched/12(trig_OUTP_40()) -> [trig_OUTP_40]
  hcu_main_sched/5(trig_GetDID()) -> [trig_GetDID]
  hcu_main_sched/10(trig_INP_20()) -> [trig_INP_20]
  APP/10 -> OUTP/9, [BSCP_outputs]
  INP/11 -> APP/11
  hcu_main_sched/6(trig_HAL_IN_10()) -> [trig_HAL_IN_10]
  Constant5/1 -> hcu_main_sched/1(VHAL_FusionSchedReq_flg)
  [trig_HAL_IN_10] -> HAL_IN/Trigger
  HAL_IN/1 -> INP/1
  INP/13 -> APP/13
  INP/12 -> APP/12
  INP/8 -> APP/8
  [trig_APP_30] -> APP/Trigger
  hcu_main_sched/15(trig_HAL_OUTAFTER_50_1()) -> [trig_HAL_OUTAFTER_50_1]
  hcu_main_sched/4(trig_GetNMID()) -> [trig_GetNMID]
  hcu_main_sched/1(trig_Read_NVM_00()) -> [trig_Read_NVM_00]
  [BHAL_APM_outputs] -> INP/10
  hcu_main_sched/13(trig_OUTP_AFTER_40_1()) -> [trig_OUTP_AFTER_40_1]
  [BHAL_DDM_outputs] -> INP/12
  HAL_IN/2 -> [BHAL_CAN2_outputs], INP/2
  INP/7 -> APP/7
  INP/10 -> APP/10
  hcu_main_sched/14(trig_HAL_OUT_50()) -> [trig_HAL_OUT_50]
  [BHAL_IMU_outputs] -> INP/13
  [trig_OUTP_40] -> OUTP/Trigger
  hcu_main_sched/16(trig_J1939TP_60()) -> [trig_J1939TP_60]
  HAL_IN/3 -> INP/3
  [trig_HAL_OUT_50] -> HAL_OUT/Trigger
  hcu_main_sched/7(trig_HAL_CDD_10_1()) -> [trig_HAL_CDD_10_1]
  INP/2 -> APP/2
  hcu_main_sched/11(trig_APP_30()) -> [trig_APP_30]
  INP/9 -> APP/9
  INP/4 -> APP/4
  [BSCP_outputs] -> HAL_OUT/2
  hcu_main_sched/8(trig_HAL_DKC_10_2()) -> [trig_HAL_DKC_10_2]
  hcu_main_sched/3(trig_WDG()) -> [trig_WDG]
  HAL_IN/4 -> [BHAL_CAN4_outputs], INP/4
  [BHAL_DKC_outputs] -> INP/11
  INP/3 -> APP/3
  [BHAL_TPMS_outputs] -> INP/8
  OUTP/1 -> [BOUTP_outputs], HAL_OUT/1
  hcu_main_sched/2(trig_ReadIMUOffset_00()) -> [trig_ReadIMUOffset_00]
  HAL_IN/5 -> INP/5
  HAL_IN/6 -> INP/6
  [s8_AcoreReadyToSleep] -> HAL_OUT/3
  [BHAL_SYS_outputs] -> INP/9
  INP/6 -> APP/6
  [trig_INP_20] -> INP/Trigger
  [BHAL_GPIO_outputs] -> INP/7
  hcu_main_sched/9(trig_HAL_DKC_10_3()) -> [trig_HAL_DKC_10_3]
  R_CAN1_DCDC_Status_1_CAN1_SG_DCDC_Status_1_read/1 -> HAL_IN/1
  R_CAN1_DCDC_Status_2_CAN1_SG_DCDC_Status_2_read/1 -> HAL_IN/2
  R_CAN1_EAC_Status_1_CAN1_SG_EAC_Status_1_read/1 -> HAL_IN/3
  R_CAN1_EBC1_CAN1_SG_EBC1_read/1 -> HAL_IN/4
  R_CAN1_PDU_Status_1_CAN1_SG_PDU_Status_1_read/1 -> HAL_IN/10
  R_CAN5_TBOX1_CAN5_SG_TBOX1_read/1 -> HAL_IN/37
  R_CAN5_TBOX2_CAN5_SG_TBOX2_read/1 -> HAL_IN/38
  R_CAN5_TBOX3_CAN5_SG_TBOX3_read/1 -> HAL_IN/39
  R_CAN7_Door_Fr1_CAN7_SG_Door_Fr1_read/1 -> HAL_IN/40
  HAL_OUT/1 -> P_CAN1_GW1_C1000_1_CAN1_SG_GW1_C1000_1_write/1
  HAL_OUT/2 -> P_CAN2_FD2_CE100_0_CAN2_SG_FD2_CE100_0_write/1
  HAL_OUT/3 -> P_CAN2_FD2_CE100_1_CAN2_SG_FD2_CE100_1_write/1
  HAL_OUT/4 -> P_CAN2_FD2_CE200_1_CAN2_SG_FD2_CE200_1_write/1
  HAL_OUT/5 -> P_CAN3_FD3_BCM1_CAN3_SG_FD3_BCM1_write/1
  HAL_OUT/6 -> P_CAN3_FD3_THCM2_CAN3_SG_FD3_THCM2_write/1
  HAL_OUT/7 -> P_CAN3_FD3_V2L1_CAN3_SG_FD3_V2L1_write/1
  HAL_OUT/8 -> P_CAN3_GW3_CE100_0_CAN3_SG_GW3_CE100_0_write/1
  HAL_OUT/9 -> P_CAN4_FD4_CE100_1_CAN4_SG_FD4_CE100_1_write/1
  HAL_OUT/10 -> P_CAN4_FD4_CE100_3_CAN4_SG_FD4_CE100_3_write/1
  HAL_OUT/11 -> P_CAN4_FD4_CE200_0_CAN4_SG_FD4_CE200_0_write/1
  HAL_OUT/12 -> P_CAN4_GW4_CE100_0_CAN4_SG_GW4_CE100_0_write/1
  HAL_OUT/13 -> P_CAN5_FD5_CE100_0_CAN5_SG_FD5_CE100_0_write/1
  HAL_OUT/14 -> P_CAN5_FD5_Debug1_CAN5_SG_FD5_Debug1_write/1
  HAL_OUT/15 -> P_CAN5_GW5_CE100_0_CAN5_SG_GW5_CE100_0_write/1
  HAL_OUT/16 -> P_CAN7_FD7_CE100_0_CAN7_SG_FD7_CE100_0_write/1
  HAL_OUT/17 -> P_CAN7_FD7_CE100_1_CAN7_SG_FD7_CE100_1_write/1
  HAL_OUT/18 -> IRV_ms10_CAN1_SG_EMRC1_write/1
  HAL_OUT/19 -> IRV_ms10_CAN1_SG_VCU_PDU_Demand_1_write/1
  HAL_OUT/20 -> IRV_ms10_CAN2_SG_GW2_C10_0_write/1
  HAL_OUT/21 -> IRV_ms10_CAN3_SG_FD3_VCU0_write/1
  HAL_OUT/22 -> IRV_ms10_CAN3_SG_FD3_VCU2_write/1
  HAL_OUT/23 -> IRV_ms10_CAN3_SG_FD3_VCU2_toNIDEC_write/1
  HAL_OUT/24 -> IRV_ms10_CAN3_SG_FD3_VCU5_write/1
  HAL_OUT/25 -> IRV_ms100_CAN1_SG_CCVS_write/1
  HAL_OUT/26 -> IRV_ms100_CAN1_SG_FD1_C100_1_write/1
  HAL_OUT/27 -> IRV_ms100_CAN1_SG_FD1_C100_2_write/1
  HAL_OUT/28 -> IRV_ms100_CAN1_SG_FD1_C100_3_write/1
  HAL_OUT/29 -> IRV_ms100_CAN1_SG_FD1_CE100_1_write/1
  HAL_OUT/30 -> IRV_ms100_CAN1_SG_GW1_C100_4_write/1
  HAL_OUT/31 -> IRV_ms100_CAN2_SG_FD2_C200_1_write/1
  HAL_OUT/32 -> IRV_ms100_CAN3_SG_FD3_THCM1_write/1
  HAL_OUT/33 -> IRV_ms100_CAN4_SG_FD4_C100_0_write/1
  HAL_OUT/34 -> IRV_ms20_CAN2_SG_FD2_C20_0_write/1
  HAL_OUT/35 -> IRV_ms250_CAN1_SG_EEC3_write/1
  HAL_OUT/36 -> IRV_ms50_CAN1_SG_EEC2_write/1
  HAL_OUT/37 -> IRV_ms50_CAN1_SG_ETC2_write/1
  HAL_OUT/38 -> IRV_ms5000_CAN2_SG_FD2_Version_write/1
  HAL_OUT/39 -> IRV_ms80_CAN1_SG_ETC1_write/1
  HAL_OUT/40 -> IRV_E2E_CAN3_SG_FD3_VCU1_write/1
  HAL_OUT/41 -> IRV_E2E_CAN3_SG_FD3_VCU1_toNIDEC_write/1
  HAL_OUT/42 -> IRV_E2E_CAN4_SG_FD4_CE100_0_write/1
  HAL_OUT/50 -> [VOUTP_IVIRST_flg]
  HAL_OUT/49 -> [VOUTP_FdcSlpTime_sec]
  HAL_OUT/51 -> [E2E_CAN3_VCU1_Trigger]
  HAL_OUT/48 -> [VOUTP_FdcSlpReqRisingEdge_flg]
  HAL_OUT/52 -> [E2E_CAN3_VCU1_toNIDEC_Trigger]
  HAL_OUT/54 -> [CONFGEM1_BAM_Trigger]
  HAL_OUT/55 -> [CONFGEM1_DT_Trigger]
  HAL_OUT/47 -> [VOUTP_NvWriteReqRisingEdge_flg]
  HAL_OUT/53 -> [E2E_CAN4_VCU1_Trigger]
  HAL_OUT/43 -> [J1939_CAN1_SG_CFGEM1_BAM]
  HAL_OUT/44 -> [J1939_CAN1_SG_CFGEM1_DT]
  HAL_OUT/46 -> [VOUTP_SysPowerMode_enum]
  HAL_OUT/45 -> [VOUTP_NetworkReq_flg]
  [u8_GetAPS_V_Rq_EPAS_Ctrl] -> Halin_CDD/68(u8_GetAPS_V_Rq_EPAS_Ctrl)
  [u8_PwrReqOTA] -> Halin_CDD/29(VHAL_PwrReq_OTA_enum)
  Halin_CDD/4(BHAL_TPMS_outputs) -> [BHAL_TPMS_outputs]
  [u8_GetAPS_HW_Ver] -> Halin_CDD/64(u8_GetAPS_HW_Ver)
  [u8_GetAPS_DecReq_A] -> Halin_CDD/72(u8_GetAPS_DecReq_A)
  [u8_GetAPS_Rq_EPAS_Ctrl] -> Halin_CDD/69(u8_GetAPS_Rq_EPAS_Ctrl)
  [u8_GetAPS_Progress_PCT] -> Halin_CDD/61(u8_GetAPS_Progress_PCT)
  [u16_Pedal2Vol] -> Halin_CDD/10(VHAL_AccelPedal2Vol_Raw)
  [u8Array12_ApsInUssSta] -> Halin_CDD/4(APSFaultStaData)
  Halin_CDD/7(BHAL_IMU_outputs) -> [BHAL_IMU_outputs]
  [u8_GetCAAS_Sta] -> Halin_CDD/76(u8_GetCAAS_Sta)
  [trig_HAL_CDD_10_1] -> Halin_CDD/Trigger
  [u8_CAN1BusOff] -> Halin_CDD/56(VHAL_CAN1BusOff_raw)
  [u8_TrunkHanSW] -> Halin_CDD/21(VHAL_TrunkHanSW_flg)
  [u8_GetAPS_Req] -> Halin_CDD/70(u8_GetAPS_Req)
  [u16_Pedal1Ref5V] -> Halin_CDD/49(VHAL_Pedal1Ref5V_raw)
  Halin_CDD/2(BHAL_GPIO_outputs) -> [BHAL_GPIO_outputs]
  [u8_GetAPS_VMC_Req_A] -> Halin_CDD/75(u8_GetAPS_VMC_Req_A)
  [u8_BrakeSW] -> Halin_CDD/11(VHAL_BrakeSWGPIO_flg)
  [u8_DrDoorSW] -> Halin_CDD/14(VHAL_DrDoorSW_flg)
  [u8_RRDoorSW] -> Halin_CDD/16(VHAL_RRDoorSW_flg)
  [u8_GetAPS_ExitCondition] -> Halin_CDD/65(u8_GetAPS_ExitCondition)
  [u8Array4_HWID] -> Halin_CDD/24(u8_HWID_4byte)
  Halin_CDD/3(BHAL_SYS_outputs) -> [BHAL_SYS_outputs]
  [f32_GetAPS_DecReq] -> Halin_CDD/71(f32_GetAPS_DecReq)
  [f32_GetAPS_SpeedCmd] -> Halin_CDD/73(f32_GetAPS_SpeedCmd)
  [u8_TPMSDataInSta] -> Halin_CDD/38(TPMS_DataIn_flg)
  Halin_CDD/1(BHAL_APM_outputs) -> [BHAL_APM_outputs]
  [u8_GetAPS_SW_Ver] -> Halin_CDD/63(u8_GetAPS_SW_Ver)
  [VHAL_NetworkReqCalled_flg] -> Halin_CDD/51(VHAL_NetworkReqCalled_flg)
  [u8_ApsInSysFailSta] -> Halin_CDD/7(StaFSyaIn)
  [u8_GetAPS_RQ_Display] -> Halin_CDD/62(u8_GetAPS_RQ_Display)
  [u8_CAN5BusOff] -> Halin_CDD/60(VHAL_CAN5BusOff_raw)
  [s8_AcoreReadyToSleep] -> Halin_CDD/32(VHAL_AcoreReadyToSlp_flg)
  [u8_GetAPS_Sta_System] -> Halin_CDD/67(u8_GetAPS_Sta_System)
  [u8_AnyNMID] -> Halin_CDD/27(VHAL_AnyNMID_flg)
  [u8_ApsInSysMode] -> Halin_CDD/8(ModOperationIn)
  [u16_Pedal2Ref5V] -> Halin_CDD/50(VHAL_Pedal2Ref5V_raw)
  [u16_AuxBattVol100mV] -> Halin_CDD/48(VHAL_AuxBattVolmV_100mV)
  [u16_Pedal1Vol] -> Halin_CDD/9(VHAL_AccelPedal1Vol_Raw)
  Constant6/1 -> Halin_CDD/25(GetSWID_status)
  [u8_CAN4BusOff] -> Halin_CDD/59(VHAL_CAN4BusOff_raw)
  [u8_AllowMovThdOTA] -> Halin_CDD/30(VHAL_AllowMovThd_OTA_enum)
  [u8_IMUOffsetValSta] -> Halin_CDD/45(VHAL_IMUOffsetValSta_flg)
  [u8_HazardSW] -> Halin_CDD/19(VHAL_HazardSW_flg)
  [u8_EvccAplusPwrUpReq] -> Halin_CDD/31(VHAL_EvccAplusPwrUpReq_flg)
  [u8_ApsInPASChime] -> Halin_CDD/5(ChimeIn)
  [u8Array30_SWID] -> Halin_CDD/26(GetSWID_data)
  [BHAL_CAN4_outputs] -> Halin_CDD/41(BHAL_CAN4_outputs)
  [u8_CrashSignal] -> Halin_CDD/23(VHAL_CrashSignalGPIO_flg)
  [u8_CAN2BusOff] -> Halin_CDD/57(VHAL_CAN2BusOff_raw)
  [f32_GetAPS_Angle_Target] -> Halin_CDD/66(f32_GetAPS_Angle_Target)
  [u8Array8_ApsInLevel] -> Halin_CDD/3(APSLevelData)
  Halin_CDD/5(BHAL_SYSTPMS_outputs) -> [BHAL_SYSTPMS_outputs]
  [u8_HoodSW] -> Halin_CDD/12(VHAL_HoodSW_flg)
  [u8Array256_NvmReadArray] -> Halin_CDD/35(HAL_NvmReadData_raw)
  [u8_BootReason] -> Halin_CDD/52(VHAL_PmicBootReason_enum)
  [u8_GetCAAS_VMC_Req_A] -> Halin_CDD/77(u8_GetCAAS_VMC_Req_A)
  [u8_TailgateSW] -> Halin_CDD/13(VHAL_TailgateSW_flg)
  [u8_DidStaDKC] -> Halin_CDD/36(VHAL_DIDVCUKeyReadSta_flg)
  [u8_RLDoorSW] -> Halin_CDD/17(VHAL_RLDoorSW_flg)
  [u8Array9_TPMSData] -> Halin_CDD/39(TPMS_RawData)
  [u8Array8_DidDataDKC] -> Halin_CDD/37(VHAL_GetDIDVCUKey_enum)
  [u8_GetAPS_ShftPosnReq] -> Halin_CDD/74(u8_GetAPS_ShftPosnReq)
  [u8_DidDataXWD] -> Halin_CDD/34(VHAL_DidXWDData_enum)
  [u8_ClearDTCcmd] -> Halin_CDD/42(VHAL_ClearDTCcmd_flg)
  [u8_CAN3BusOff] -> Halin_CDD/58(VHAL_CAN3BusOff_raw)
  [u8_AcoreRebootCmd] -> Halin_CDD/55(VHAL_AcoreRebootCmd_raw)
  [u8_SeatSW] -> Halin_CDD/22(VHAL_SeatSW_flg)
  [u8_CurrentNMState] -> Halin_CDD/28(VHAL_CurrentNmState_enum)
  [u8_BrakeLamp] -> Halin_CDD/20(VHAL_BrakeLampSW_flg)
  [u32_WISR] -> Halin_CDD/53(VHAL_WisrBootReason_raw32)
  [u8_NvmProtectSta] -> Halin_CDD/47(VHAL_NvmProtectSta_flg)
  [u8Array8_PasInDist] -> Halin_CDD/1(PASDistanceData)
  [BHAL_DIDGetData_raw] -> Halin_CDD/54(BHAL_DIDGetData_raw)
  [u8_DidStaXWD] -> Halin_CDD/33(VHAL_DidXWDSta_flg)
  [s16_IMUSixAxisVal] -> Halin_CDD/44(VHAL_IMUSixAxisVal_raw)
  [u8_PsDoorSW] -> Halin_CDD/15(VHAL_PsDoorSW_flg)
  Halin_CDD/6(BHAL_DDM_outputs) -> [BHAL_DDM_outputs]
  [u8_CTDSW] -> Halin_CDD/18(VHAL_CentralDoorLockSW_flg)
  [u16Array4_ApsInDist] -> Halin_CDD/2(APSDistanceData)
  Halin_CDD/8(Enable_decrypt) -> [Enable_decrypt]
  [BHAL_CAN2_outputs] -> Halin_CDD/40(BHAL_CAN2_outputs)
  [u8_ApsInSensorLayout] -> Halin_CDD/6(SNSRLayoutIn)
  [u8_IMUSixAxisValSta] -> Halin_CDD/46(VHAL_IMUSixAxisValSta_flg)
  [s16_IMUOffsetVal] -> Halin_CDD/43(VHAL_IMUOffsetVal_raw)
  OUTP_AFTER/10(DTC_Array) -> Goto108/1
  OUTP_AFTER/3(ApsOut_SetFrSensorOnCmd) -> [u8_ApsOutSetFrSensorOnCmd]
  OUTP_AFTER/1(ApsOut_GearPosnSig) -> [u8_ApsOutGearPosnSig]
  [BOUTP_outputs] -> OUTP_AFTER/1(BOUTP_outputs)
  [trig_OUTP_AFTER_40_1] -> OUTP_AFTER/Trigger
  OUTP_AFTER/11(BOUTP_DIDSetData_outputs) -> [BOUTP_DIDSetData_outputs]
  OUTP_AFTER/2(ApsOut_SendChrgPlugStaSig) -> [u8_ApsOutSendChrgPlugSta]
  OUTP_AFTER/7(HAL_NvmWriteData_raw) -> [u8Array256_NvmWriteArray]
  [BHAL_SYS_outputs] -> OUTP_AFTER/3(BHAL_SYS_outputs)
  OUTP_AFTER/6(ApsOut_VehSpdSig) -> [f32_ApsOutVehSpdSig]
  OUTP_AFTER/4(ApsOut_SetFrSensorSwTOCmd) -> [u8_ApsOutSetFrSensorSwTOCmd]
  OUTP_AFTER/5(ApsOut_SetVehSpdTOCmd) -> [u8_ApsOutSetVehSpdTOCmd]
  [BHAL_SYSTPMS_outputs] -> OUTP_AFTER/2(BHAL_SYSTPMS_outputs)
  OUTP_AFTER/9(Header_Array) -> Goto103/1
  OUTP_AFTER/8(DTC_Trigger) -> Goto116/1
  [BHAL_CAN4_outputs] -> Subsystem2/3(BHAL_CAN4_outputs)
  [Enable_decrypt] -> Subsystem2/1(Enable_Decrypt)
  [u8Array16_ResultData] -> Subsystem2/2(u8Array16_ResultData)
  [trig_HAL_DKC_10_3] -> Subsystem2/Trigger
  Subsystem2/1(BHAL_DKC_outputs) -> [BHAL_DKC_outputs]
  [trig_HAL_DKC_10_2] -> Subsystem/Trigger
  Halin_CDD/9(AESKey) -> Subsystem/1(In1)
  Halin_CDD/10(DKCRawData) -> Subsystem/2(In2)
  Subsystem/1(Out1) -> [u8Array16_ResultData]
  Data Type Conversion5/1 -> Subsystem1/1(In1)
  [VOUTP_IVIRST_flg] -> Data Type Conversion5/1
  Bus Selector1/1 -> R_HALOUTCDD_CSOP_SetAcoreRebootCmdACK/Enable  "<VOUTP_AcoreRebootCmdACK_flg>"
  [BOUTP_outputs] -> Bus Selector1/1
  Bus Selector/1 -> R_UDSCDD_CSOP_DdmRestartOperationCycle/Enable  "<VOUTP_EnterNewOperCyc_flg>"
  From129/1 -> Bus Selector/1
  Ground10/1 -> Subsystem3/Enable, Subsystem1/Enable
  Cast To Boolean/1 -> Subsystem4/1(Trig_BAM)
  Cast To Boolean1/1 -> Subsystem4/2(Trig_DT)
  [CONFGEM1_DT_Trigger] -> Unit Delay5/1
  [trig_J1939TP_60] -> Subsystem4/Trigger
  Unit Delay4/1 -> Cast To Boolean/1
  Unit Delay5/1 -> Cast To Boolean1/1
  [CONFGEM1_BAM_Trigger] -> Unit Delay4/1
  Subsystem5/1(Out1) -> [BHAL_DIDGetData_raw]
  [trig_GetDID] -> Subsystem5/Trigger
  [BOUTP_DIDSetData_outputs] -> Subsystem5/1(In1)
  R_CAN2_METER1_CAN2_SG_METER1_read/1 -> HAL_IN/11
  R_CAN2_IVI1_CAN2_SG_IVI1_read/1 -> HAL_IN/12
  R_CAN3_BMS6_CAN3_SG_BMS6_read/1 -> HAL_IN/17
  R_CAN3_BMS8_CAN3_SG_BMS8_read/1 -> HAL_IN/18
  R_CAN3_CCU2_CAN3_SG_CCU2_read/1 -> HAL_IN/19
  R_CAN3_MCU_B_R1_CAN3_SG_MCU_B_R1_read/1 -> HAL_IN/20
  R_CAN3_BMS5_CAN3_SG_BMS5_read/1 -> HAL_IN/23
  R_CAN2_IVI2_CAN2_SG_IVI2_read/1 -> HAL_IN/13
  R_CAN3_Shifter1_CAN3_SG_Shifter1_read/1 -> HAL_IN/21
  R_CAN3_BMS4_CAN3_SG_BMS4_read/1 -> HAL_IN/22
  R_CAN2_IVI_P20_0_CAN2_SG_IVI_P20_0_read/1 -> HAL_IN/14
  R_CAN3_BMS1_CAN3_SG_BMS1_read/1 -> HAL_IN/15
  R_CAN3_BMS3_CAN3_SG_BMS3_read/1 -> HAL_IN/16
  R_CAN3_CCU1_CAN3_SG_CCU1_read/1 -> HAL_IN/24
  R_CAN3_MCU_B_R2_CAN3_SG_MCU_B_R2_read/1 -> HAL_IN/25
  R_CAN4_DKC1_CAN4_SG_DKC1_read/1 -> HAL_IN/33
  R_CAN4_ZONE_FR1_CAN4_SG_ZONE_FR1_read/1 -> HAL_IN/34
  R_CAN4_ZONE_DR_VCU_CAN4_SG_ZONE_DR_VCU_read/1 -> HAL_IN/32
  R_CAN4_ZONE_FR_VCU_CAN4_SG_ZONE_FR_VCU_read/1 -> HAL_IN/35
  R_CAN4_zGW_APTC1_CAN4_SG_zGW_APTC1_read/1 -> HAL_IN/26
  R_CAN4_zGW_CANFr1_CAN4_SG_zGW_CANFr1_read/1 -> HAL_IN/27
  R_CAN4_zGW_LINDr1_CAN4_SG_zGW_LINDr1_read/1 -> HAL_IN/28
  R_CAN4_DKC2_CAN4_SG_DKC2_read/1 -> HAL_IN/29
  R_CAN4_Z24_C1000_0_CAN4_SG_Z24_C1000_0_read/1 -> HAL_IN/30
  R_CAN4_Z24_CE100_0_CAN4_SG_Z24_CE100_0_read/1 -> HAL_IN/31
  R_CAN4_ZONE_DR1_CAN4_SG_ZONE_DR1_read/1 -> HAL_IN/36
  [BOUTP_outputs] -> Subsystem3/1(BOUTP_outputs)
  R_CAN1_EBC5_CAN1_SG_EBC5_read/1 -> HAL_IN/5
  R_CAN1_EHPS_Status_1_CAN1_SG_EHPS_Status_1_read/1 -> HAL_IN/6
  R_CAN1_EMC1_EM1_CAN1_SG_EMC1_EM1_read/1 -> HAL_IN/7
  R_CAN1_EPB1_CAN1_SG_EPB1_read/1 -> HAL_IN/8
  R_CAN1_EBC2_CAN1_SG_EBC2_read/1 -> HAL_IN/9
  APP/1 -> OUTP/1
  APP/2 -> OUTP/2
  APP/3 -> OUTP/3
  APP/5 -> OUTP/4
  APP/6 -> OUTP/5
  APP/7 -> OUTP/6
  APP/8 -> OUTP/7
  APP/9 -> OUTP/8
  APP/11 -> OUTP/10
  APP/12 -> OUTP/11
  APP/13 -> OUTP/12
  APP/14 -> OUTP/13
  APP/15 -> OUTP/14
  APP/16 -> OUTP/15
  APP/17 -> OUTP/16
  APP/4 -> Terminator/1

== system SWC_FDC_type/run_SWC_FDC_Tx_100ms_sys ==
  IRV_ms100_CAN1_SG_CCVS_read : Inport
  IRV_ms100_CAN1_SG_FD1_C100_1_read : Inport  Port=2
  IRV_ms100_CAN1_SG_FD1_C100_2_read : Inport  Port=3
  IRV_ms100_CAN1_SG_FD1_C100_3_read : Inport  Port=4
  IRV_ms100_CAN1_SG_FD1_CE100_1_read : Inport  Port=5
  IRV_ms100_CAN1_SG_GW1_C100_4_read : Inport  Port=6
  IRV_ms100_CAN2_SG_FD2_C200_1_read : Inport  Port=7
  IRV_ms100_CAN3_SG_FD3_THCM1_read : Inport  Port=8
  IRV_ms100_CAN4_SG_FD4_C100_0_read : Inport  Port=9
  function : TriggerPort  TriggerType=function-call  VariantControl=(inherit)  SampleTimeType=periodic  SampleTime=-1
  P_CAN1_CCVS_CAN1_SG_CCVS_write : Outport
  P_CAN1_FD1_C100_1_CAN1_SG_FD1_C100_1_write : Outport  Port=2
  P_CAN1_FD1_C100_2_CAN1_SG_FD1_C100_2_write : Outport  Port=3
  P_CAN1_FD1_C100_3_CAN1_SG_FD1_C100_3_write : Outport  Port=4
  P_CAN1_FD1_CE100_1_CAN1_SG_FD1_CE100_1_write : Outport  Port=5
  P_CAN1_GW1_C100_4_CAN1_SG_GW1_C100_4_write : Outport  Port=6
  P_CAN2_FD2_C200_1_CAN2_SG_FD2_C200_1_write : Outport  Port=7
  P_CAN3_FD3_THCM1_CAN3_SG_FD3_THCM1_write : Outport  Port=8
  P_CAN4_FD4_C100_0_CAN4_SG_FD4_C100_0_write : Outport  Port=9
  wires:
  IRV_ms100_CAN1_SG_CCVS_read/1 -> P_CAN1_CCVS_CAN1_SG_CCVS_write/1
  IRV_ms100_CAN1_SG_FD1_C100_1_read/1 -> P_CAN1_FD1_C100_1_CAN1_SG_FD1_C100_1_write/1
  IRV_ms100_CAN1_SG_FD1_C100_2_read/1 -> P_CAN1_FD1_C100_2_CAN1_SG_FD1_C100_2_write/1
  IRV_ms100_CAN1_SG_FD1_C100_3_read/1 -> P_CAN1_FD1_C100_3_CAN1_SG_FD1_C100_3_write/1
  IRV_ms100_CAN1_SG_FD1_CE100_1_read/1 -> P_CAN1_FD1_CE100_1_CAN1_SG_FD1_CE100_1_write/1
  IRV_ms100_CAN1_SG_GW1_C100_4_read/1 -> P_CAN1_GW1_C100_4_CAN1_SG_GW1_C100_4_write/1
  IRV_ms100_CAN2_SG_FD2_C200_1_read/1 -> P_CAN2_FD2_C200_1_CAN2_SG_FD2_C200_1_write/1
  IRV_ms100_CAN3_SG_FD3_THCM1_read/1 -> P_CAN3_FD3_THCM1_CAN3_SG_FD3_THCM1_write/1
  IRV_ms100_CAN4_SG_FD4_C100_0_read/1 -> P_CAN4_FD4_C100_0_CAN4_SG_FD4_C100_0_write/1
